simulink model "plantaEstacionamento"  (R2023b)
settings: Solver=VariableStepAuto  StartTime=0.0  StopTime=1e8  RelTol=1e-3
values from neighbouring files (symbols this model uses):
  controlador = projetarControladorAnalitico()    [main.m]    (also in otimizacao.m; otimizacaoCmaes.m = projetarControladorAnalitico(requisitos, planta))
  planta = obterPlantaProjeto()    [avaliarControladorAnalitico.m]    (also in calcularCusto.m = obterPlanta(); main.m; otimizacao.m; otimizacaoCmaes.m = obterPlanta())
libraries: simulink x1
settings Model: Creator=gabri  LastModifiedBy=gubid

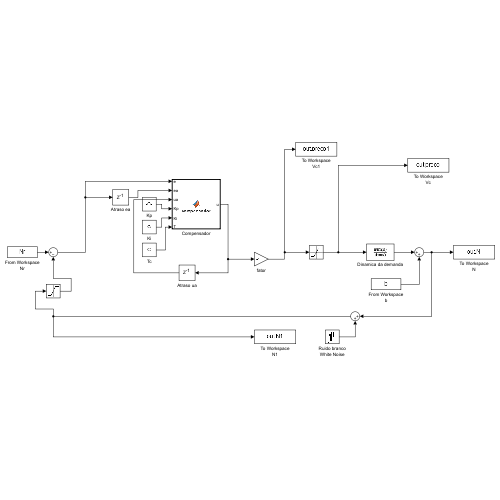
[thumbnail: Simulink's stored preview of the top-level diagram]
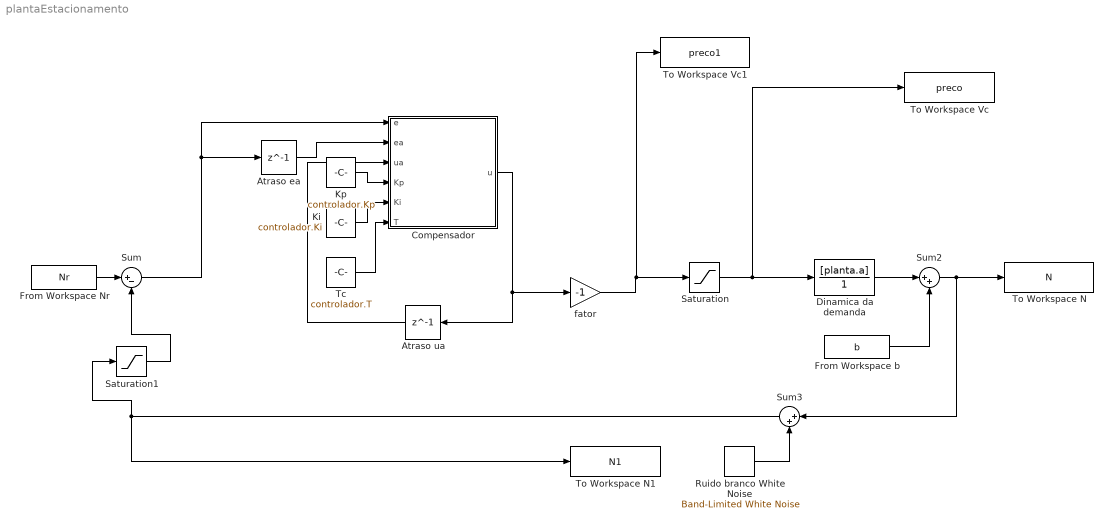
== system plantaEstacionamento ==
  Atraso ea : Delay  DelayLength=1  InitialCondition=0  SampleTime=controlador.T
  Atraso ua : Delay  DelayLength=1  InitialCondition=0  SampleTime=controlador.T
  Compensador : MATLAB Function  TreatAsAtomicUnit=on  SystemSampleTime=controlador.T
  Dinamica da demanda : TransferFcn  Numerator=[planta.a]  Denominator=[1]
  From Workspace Nr : FromWorkspace  VariableName=Nr
  From Workspace b : FromWorkspace  VariableName=b  OutDataTypeStr=double
  Ki : Constant  Value=controlador.Ki
  Kp : Constant  Value=controlador.Kp
  Ruido branco White Noise : simulink/Sources/Band-Limited White Noise  Cov=[0.1]  Ts=864000  seed=[23341]
  Saturation : Saturate  UpperLimit=inf  LowerLimit=0
  Saturation1 : Saturate  UpperLimit=1  LowerLimit=0
  Sum : Sum  Inputs=|+-
  Sum2 : Sum  Inputs=|++
  Sum3 : Sum  Inputs=|++
  Tc : Constant  Value=controlador.T
  To Workspace N : ToWorkspace  VariableName=N  SaveFormat=Structure With Time  SampleTime=3600
  To Workspace N1 : ToWorkspace  VariableName=N1  SaveFormat=Structure With Time  SampleTime=3600
  To Workspace Vc : ToWorkspace  VariableName=preco  SaveFormat=Structure With Time  SampleTime=3600
  To Workspace Vc1 : ToWorkspace  VariableName=preco1  SaveFormat=Structure With Time  SampleTime=3600
  fator : Gain  Gain=-1
  wires:
  Dinamica da demanda/1 -> Sum2/1
  From Workspace Nr/1 -> Sum/1
  Compensador/1(u) -> fator/1, Atraso ua/1
  From Workspace b/1 -> Sum2/2
  Sum2/1 -> Sum3/1, To Workspace N/1
  Sum3/1 -> Saturation1/1, To Workspace N1/1
  Ruido branco White Noise/1 -> Sum3/2
  Tc/1 -> Compensador/6(T)
  Sum/1 -> Compensador/1(e), Atraso ea/1
  Ki/1 -> Compensador/5(Ki)
  Atraso ua/1 -> Compensador/3(ua)
  Atraso ea/1 -> Compensador/2(ea)
  Kp/1 -> Compensador/4(Kp)
  fator/1 -> To Workspace Vc1/1, Saturation/1
  Saturation/1 -> To Workspace Vc/1, Dinamica da demanda/1
  Saturation1/1 -> Sum/2

== matlab function plantaEstacionamento/Compensador ==
  data: e input; u output; ea input; ua input; Kp input; Ki input; T input
function u = compensador(e, ea, ua, Kp, Ki, T)
% u = compensador(e, ea, ua, Kp, Ki, T, Vmax)
% Implementa o compensador PI discreto.
% Entradas:
% e: erro atual e[k].
% ea: erro anterior e[k-1].
% ua: comando anterior u[k-1].
% Kp: ganho proporcional.
% Ki: ganho integrativo.
% T: tempo de amostragem.
% Vmax: limite de tensao.
% Saidas:
% u: comando atual u[k].

u = ua + (Kp + Ki*T/2)*e + (-Kp + Ki*T/2)*ea; % Implementar compensador

end
